simulink model "euler_attitude_control"  (Simulink 7.1)
settings: Solver=ode45  StartTime=0.0  StopTime=30.0  MaxStep=.01  RelTol=1e-3
libraries: aerolib6dof2 x1
settings Model: Creator=Administrator  LastModifiedBy=Administrator

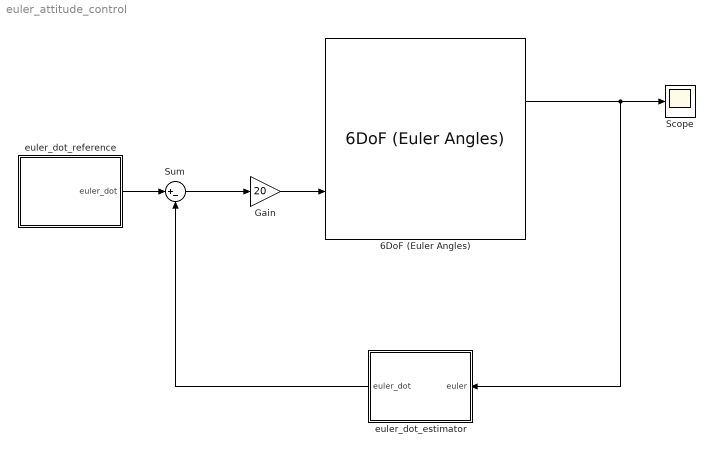
== system euler_attitude_control ==
  6DoF (Euler Angles) : aerolib6dof2/6DoF (Euler Angles)  SystemSampleTime=-1  units=Metric (MKS)  mtype=Fixed  rep=Euler Angles  xme_0=[0 0 0]  Vm_0=[0 0 0]  eul_0=[0 0 0]  pm_0=[0 0 0]  mass_0=1.8263  mass_e=0.5  mass_f=2.0  inertia=diag([0.02759 0.02771 0.04806])  inertia_e=eye(3)  inertia_f=2*eye(3)  k_quat=1.0
  Gain : Gain  Gain=20  ParameterDataType=sfix(16)  ParameterScaling=2^0  OutDataType=sfix(16)  OutScaling=2^0
  Scope : Scope
      settings: YMin=-22500  YMax=2500  Decimation=10
  Sum : Sum  Inputs=|+-  OutDataType=sfix(16)  OutScaling=2^0
  euler_dot_estimator : Subsystem  Orientation=left
  euler_dot_reference : Subsystem
  wires:
  6DoF (Euler Angles)/3 -> euler_dot_estimator/1(euler), Scope/1
  euler_dot_estimator/1(euler_dot) -> Sum/2
  Sum/1 -> Gain/1
  euler_dot_reference/1(euler_dot) -> Sum/1
  Gain/1 -> 6DoF (Euler Angles)/2

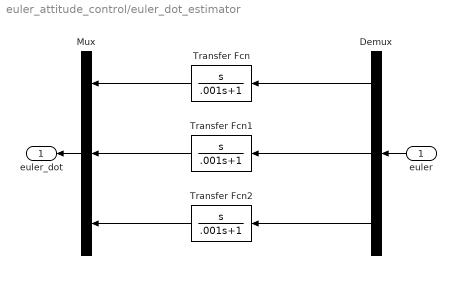
== system euler_attitude_control/euler_dot_estimator ==
  euler : Inport  Orientation=left
  Demux : Demux  Orientation=left  Outputs=3
  Mux : Mux  Orientation=left  Inputs=3
  Transfer Fcn : TransferFcn  Orientation=left  Numerator=[1 0]  Denominator=[.001 1]
  Transfer Fcn1 : TransferFcn  Orientation=left  Numerator=[1 0]  Denominator=[.001 1]
  Transfer Fcn2 : TransferFcn  Orientation=left  Numerator=[1 0]  Denominator=[.001 1]
  euler_dot : Outport  Orientation=left
  wires:
  Demux/1 -> Transfer Fcn/1
  Demux/2 -> Transfer Fcn1/1
  Demux/3 -> Transfer Fcn2/1
  Transfer Fcn/1 -> Mux/1
  Transfer Fcn1/1 -> Mux/2
  Transfer Fcn2/1 -> Mux/3
  euler/1 -> Demux/1
  Mux/1 -> euler_dot/1

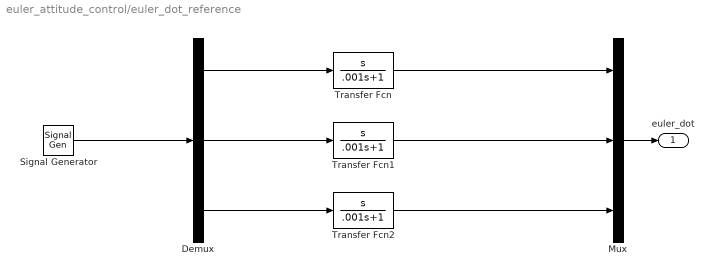
== system euler_attitude_control/euler_dot_reference ==
  Demux : Demux  Outputs=3
  Mux : Mux  Inputs=3
  Signal Generator : SignalGenerator  Amplitude=(pi*.5*58/180)*ones(3,1)  Frequency=1*ones(3,1)
  Transfer Fcn : TransferFcn  Numerator=[1 0]  Denominator=[.001 1]
  Transfer Fcn1 : TransferFcn  Numerator=[1 0]  Denominator=[.001 1]
  Transfer Fcn2 : TransferFcn  Numerator=[1 0]  Denominator=[.001 1]
  euler_dot : Outport
  wires:
  Transfer Fcn2/1 -> Mux/3
  Transfer Fcn1/1 -> Mux/2
  Transfer Fcn/1 -> Mux/1
  Demux/3 -> Transfer Fcn2/1
  Demux/2 -> Transfer Fcn1/1
  Demux/1 -> Transfer Fcn/1
  Mux/1 -> euler_dot/1
  Signal Generator/1 -> Demux/1
